simulink model "inertia2"  (R2022b)
settings: Solver=FixedStepAuto  StartTime=0.0  StopTime=t_s  FixedStep=h  RelTol=1e-3
undefined symbols (not defined in the file): J, K
libraries: simulink x1
settings Model: Creator=Claudia  LastModifiedBy=Claudia Yasar
settings SolverCC: AlgebraicLoopSolver=TrustRegion
settings DataIOCC: ReturnWorkspaceOutputs=off
settings DebuggingCC: UnconnectedInputMsg=warning  UnconnectedOutputMsg=warning  UnconnectedLineMsg=warning  SFMachineParentedDataDiag=warning  ArithmeticOperatorsInVariantConditions=warning
settings ModelReferenceCC: EnableRefExpFcnMdlSchedulingChecks=on
settings SFSimCC: CustomCodeUndefinedFunction=UseInterfaceOnly

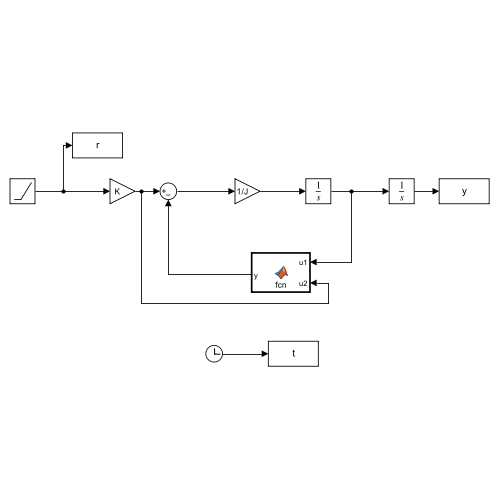
[thumbnail: Simulink's stored preview of the top-level diagram]
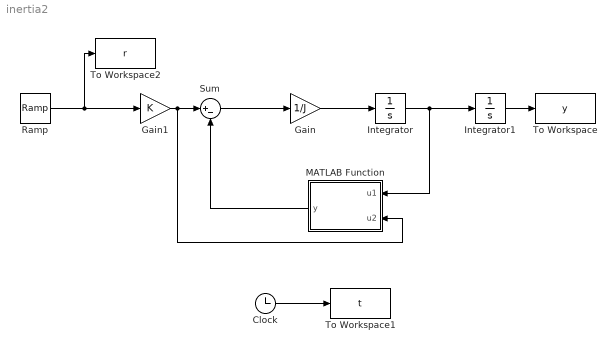
== system inertia2 ==
  Clock : Clock
  Gain : Gain  Gain=1/J
  Gain1 : Gain  Gain=K
  Integrator : Integrator
  Integrator1 : Integrator
  MATLAB Function : MATLAB Function  TreatAsAtomicUnit=on
  Ramp : simulink/Sources/Ramp  slope=1  start=0  InitialOutput=0
  Sum : Sum  Inputs=|+-
  To Workspace : ToWorkspace  VariableName=y  SampleTime=-1
      settings: OpenFcn=figure;plot(t,y);
  To Workspace1 : ToWorkspace  VariableName=t  SampleTime=-1
  To Workspace2 : ToWorkspace  VariableName=r  SampleTime=-1
      settings: OpenFcn=figure;plot(t,y);
  wires:
  Clock/1 -> To Workspace1/1
  Ramp/1 -> Gain1/1, To Workspace2/1
  Gain/1 -> Integrator/1
  Sum/1 -> Gain/1
  Integrator/1 -> MATLAB Function/1(u1), Integrator1/1
  Integrator1/1 -> To Workspace/1
  Gain1/1 -> MATLAB Function/2(u2), Sum/1
  MATLAB Function/1(y) -> Sum/2

== matlab function inertia2/MATLAB Function ==
  data: u1 input; y output; u2 input
function y = fcn(u1,u2)
stick_torque=1;
c=1;
if u2>stick_torque || u1<stick_torque
 y = c*u1;  
else
 y = u2;
end
